simulink model "Prediction_and_cost_function_FCS_MPC_6Phase_PMSM"  (R2022a)
settings: Solver=FixedStepDiscrete  StartTime=0.0  StopTime=10.0  RelTol=1e-3
values from neighbouring files (symbols this model uses):
  f_c = 100000    [MPC_params.m]
  L_d = 2e-3    (= 0.002)    [MPC_params.m]
  L_q = 6.4e-3    (= 0.0064)    [MPC_params.m]
  L_x = 3e-3    (= 0.003)    [MPC_params.m]
  L_y = L_x    (= 0.003)    [MPC_params.m]
  p = 5    [MPC_params.m]
  psi_pm = 0.19    [MPC_params.m]
  R_ph = 0.19    [MPC_params.m]
libraries: hdlsllib x5
settings Model: DataTypeOverride=Off  Creator=Andre Merx  LastModifiedBy=Andre Merx
settings SolverCC: AlgebraicLoopSolver=TrustRegion
settings DataIOCC: LimitDataPoints=on  SaveOutput=off  SaveTime=off
settings OptimizationCC: BlockReduction=off  ConditionallyExecuteInputs=off  DefaultParameterBehavior=Inlined  LifeSpan=inf
settings DebuggingCC: AlgebraicLoopMsg=error  SingleTaskRateTransMsg=error  UnconnectedInputMsg=warning  UnconnectedOutputMsg=warning  UnconnectedLineMsg=warning  AllowSymbolicDim=off  StrictBusMsg=ErrorOnBusTreatedAsVector  SFUnexpectedBacktrackingDiag=warning  SFNoUnconditionalDefaultTransitionDiag=warning  SFExecutionAtInitializationDiag=none  SFMachineParentedDataDiag=warning  ArithmeticOperatorsInVariantConditions=warning
settings HardwareCC: ProdBitPerPointer=32  ProdBitPerSizeT=32  ProdBitPerPtrDiffT=32  ProdLargestAtomicFloat=None  ProdIntDivRoundTo=Undefined  ProdEndianess=Unspecified  ProdWordSize=32  ProdHWDeviceType=ASIC/FPGA->ASIC/FPGA  ProdEqTarget=off
settings SFSimCC: SimUseLocalCustomCode=off  CustomCodeUndefinedFunction=UseInterfaceOnly
settings RTWCC: RTWUseLocalCustomCode=off
settings CodeAppCC: StateflowObjectComments=on
settings GRTTargetCC: TargetLangStandard=C89/C90 (ANSI)
settings ConfigComp: CovScope=ReferencedModels  CovMetricSettings=dw  CovSaveCumulativeToWorkspaceVar=on  CovSaveSingleToWorkspaceVar=on  CovExternalEMLEnable=off  CovSFcnEnable=off

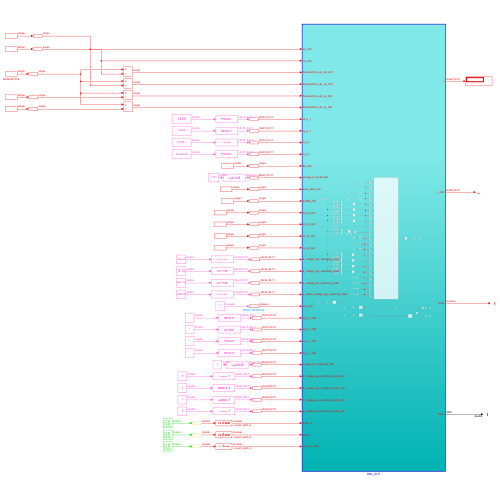
[thumbnail: Simulink's stored preview of the top-level diagram]
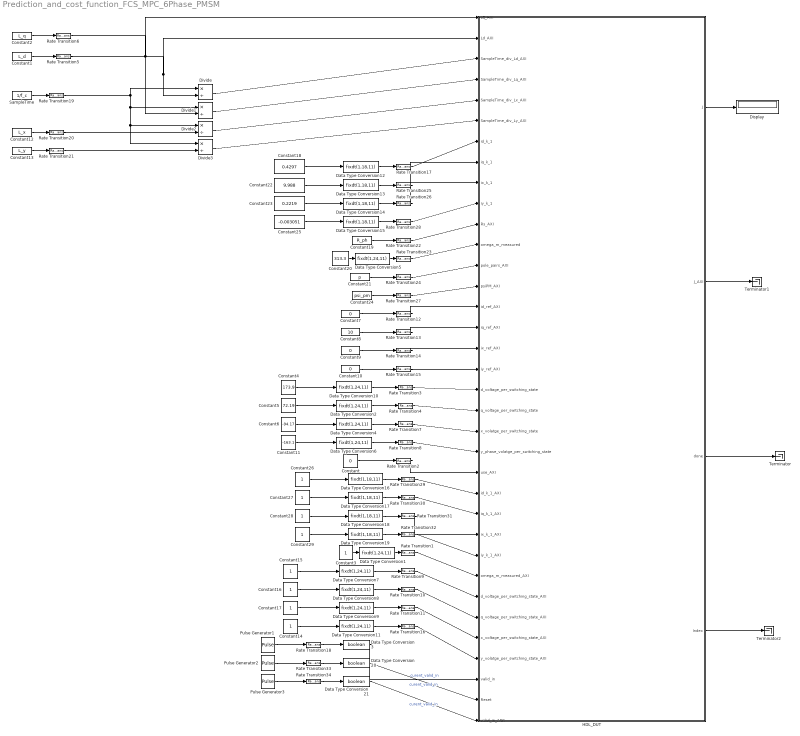
== system Prediction_and_cost_function_FCS_MPC_6Phase_PMSM ==
  Constant : Constant  Value=0  OutDataTypeStr=boolean
  Constant1 : Constant  Value=L_d  OutDataTypeStr=single  SampleTime=-1
  Constant10 : Constant  Value=0  OutDataTypeStr=single  SampleTime=-1
  Constant11 : Constant  Value=-163.1
  Constant12 : Constant  Value=L_x  OutDataTypeStr=single  SampleTime=-1
  Constant13 : Constant  Value=L_y  OutDataTypeStr=single  SampleTime=-1
  Constant{3,14..17,26..29} (9 alike) : Constant
  Constant18 : Constant  Value=0.4297
  Constant19 : Constant  Value=R_ph  OutDataTypeStr=single  SampleTime=-1
  Constant2 : Constant  Value=L_q  OutDataTypeStr=single  SampleTime=-1
  Constant20 : Constant  Value=313.3
  Constant21 : Constant  Value=p  OutDataTypeStr=single  SampleTime=-1
  Constant22 : Constant  Value=9.988
  Constant23 : Constant  Value=0.2219
  Constant24 : Constant  Value=psi_pm  OutDataTypeStr=single  SampleTime=-1
  Constant25 : Constant  Value=-0.003051
  Constant4 : Constant  Value=173.9
  Constant5 : Constant  Value=72.19
  Constant6 : Constant  Value=-94.17
  Constant7 : Constant  Value=0  OutDataTypeStr=single  SampleTime=-1
  Constant8 : Constant  Value=10  OutDataTypeStr=single  SampleTime=-1
  Constant9 : Constant  Value=0  OutDataTypeStr=single  SampleTime=-1
  Data Type Conversion{1..2,4..11} (10 alike) : DataTypeConversion  OutDataTypeStr=fixdt(1,24,11)  SaturateOnIntegerOverflow=off  RndMeth=Floor
  Data Type Conversion{12..19} (8 alike) : DataTypeConversion  OutDataTypeStr=fixdt(1,18,11)  SaturateOnIntegerOverflow=off  RndMeth=Floor
  Data Type Conversion20 : DataTypeConversion  OutDataTypeStr=boolean  SaturateOnIntegerOverflow=off  RndMeth=Floor
  Data Type Conversion21 : DataTypeConversion  OutDataTypeStr=boolean  SaturateOnIntegerOverflow=off  RndMeth=Floor
  Data Type Conversion3 : DataTypeConversion  OutDataTypeStr=boolean  SaturateOnIntegerOverflow=off  RndMeth=Floor
  Display : Display
  Divide{,1..3} (4 alike) : Product  Inputs=*/  RndMeth=Zero  SaturateOnIntegerOverflow=on
  HDL_DUT : Subsystem  TreatAsAtomicUnit=on
  Pulse Generator1 : DiscretePulseGenerator  PulseType=Time based  Period=1/f_c
  Pulse Generator2 : DiscretePulseGenerator  PulseType=Time based  Period=1/f_c
  Pulse Generator3 : DiscretePulseGenerator  PulseType=Time based  Period=1/f_c
  Rate Transition{1..34} (34 alike) : RateTransition  OutPortSampleTime=Rt
  SampleTime : Constant  Value=1/f_c  OutDataTypeStr=single  SampleTime=-1
  Terminator : Terminator
  Terminator1 : Terminator
  Terminator2 : Terminator
  wires:
  Constant7/1 -> Rate Transition12/1
  Constant9/1 -> Rate Transition14/1
  Constant8/1 -> Rate Transition13/1
  Constant10/1 -> Rate Transition15/1
  Rate Transition24/1 -> HDL_DUT/13(pole_pairs_AXI)
  Rate Transition27/1 -> HDL_DUT/14(psiPM_AXI)
  Data Type Conversion5/1 -> Rate Transition23/1
  Constant21/1 -> Rate Transition24/1
  Constant24/1 -> Rate Transition27/1
  Rate Transition23/1 -> HDL_DUT/12(omega_m_measured)
  Rate Transition22/1 -> HDL_DUT/11(Rs_AXI)
  Constant20/1 -> Data Type Conversion5/1
  Constant19/1 -> Rate Transition22/1
  Rate Transition6/1 -> HDL_DUT/1(Lq_AXI), Divide1/2
  Rate Transition5/1 -> HDL_DUT/2(Ld_AXI), Divide/2
  Constant1/1 -> Rate Transition5/1
  Constant13/1 -> Rate Transition21/1
  Rate Transition21/1 -> Divide3/2
  Constant2/1 -> Rate Transition6/1
  Constant12/1 -> Rate Transition20/1
  Rate Transition19/1 -> Divide1/1, Divide3/1, Divide2/1, Divide/1
  Rate Transition20/1 -> Divide2/2
  SampleTime/1 -> Rate Transition19/1
  Divide/1 -> HDL_DUT/3(SampleTime_div_Ld_AXI)
  Divide1/1 -> HDL_DUT/4(SampleTime_div_Lq_AXI)
  Divide2/1 -> HDL_DUT/5(SampleTime_div_Lx_AXI)
  Divide3/1 -> HDL_DUT/6(SampleTime_div_Ly_AXI)
  Rate Transition12/1 -> HDL_DUT/15(id_ref_AXI)
  Rate Transition13/1 -> HDL_DUT/16(iq_ref_AXI)
  Rate Transition14/1 -> HDL_DUT/17(ix_ref_AXI)
  Rate Transition15/1 -> HDL_DUT/18(iy_ref_AXI)
  HDL_DUT/3(done) -> Terminator/1
  HDL_DUT/2(J_AXI) -> Terminator1/1
  HDL_DUT/1(J) -> Display/1
  Data Type Conversion3/1 -> HDL_DUT/33(valid_in)  "curent_valid_in"
  Rate Transition18/1 -> Data Type Conversion3/1
  Pulse Generator1/1 -> Rate Transition18/1
  Constant3/1 -> Data Type Conversion1/1
  Data Type Conversion1/1 -> Rate Transition1/1
  Rate Transition1/1 -> HDL_DUT/28(omega_m_measured_AXI)
  Constant/1 -> Rate Transition2/1
  Rate Transition2/1 -> HDL_DUT/23(use_AXI)
  Data Type Conversion10/1 -> Rate Transition3/1
  Rate Transition3/1 -> HDL_DUT/19(d_voltage_per_switching_state)
  Data Type Conversion2/1 -> Rate Transition4/1
  Rate Transition4/1 -> HDL_DUT/20(q_voltage_per_switching_state)
  Data Type Conversion4/1 -> Rate Transition7/1
  Rate Transition7/1 -> HDL_DUT/21(x_volatge_per_switching_state)
  Data Type Conversion6/1 -> Rate Transition8/1
  Rate Transition8/1 -> HDL_DUT/22(y_phase_volatge_per_switching_state)
  Constant4/1 -> Data Type Conversion10/1
  Constant5/1 -> Data Type Conversion2/1
  Constant6/1 -> Data Type Conversion4/1
  Constant11/1 -> Data Type Conversion6/1
  Constant17/1 -> Data Type Conversion9/1
  Constant15/1 -> Data Type Conversion7/1
  Constant14/1 -> Data Type Conversion11/1
  Rate Transition16/1 -> HDL_DUT/32(y_volatge_per_switching_state_AXI)
  Constant16/1 -> Data Type Conversion8/1
  Rate Transition10/1 -> HDL_DUT/30(q_voltage_per_switching_state_AXI)
  Rate Transition11/1 -> HDL_DUT/31(x_voltage_per_switching_state_AXI)
  Data Type Conversion8/1 -> Rate Transition10/1
  Data Type Conversion9/1 -> Rate Transition11/1
  Data Type Conversion11/1 -> Rate Transition16/1
  Data Type Conversion7/1 -> Rate Transition9/1
  Rate Transition9/1 -> HDL_DUT/29(d_voltage_per_switching_state_AXI)
  Data Type Conversion12/1 -> Rate Transition17/1
  Rate Transition17/1 -> HDL_DUT/7(id_k_1)
  Data Type Conversion13/1 -> Rate Transition25/1
  Rate Transition25/1 -> HDL_DUT/8(iq_k_1)
  Data Type Conversion14/1 -> Rate Transition26/1
  Rate Transition26/1 -> HDL_DUT/9(ix_k_1)
  Data Type Conversion15/1 -> Rate Transition28/1
  Rate Transition28/1 -> HDL_DUT/10(iy_k_1)
  Constant18/1 -> Data Type Conversion12/1
  Constant22/1 -> Data Type Conversion13/1
  Constant23/1 -> Data Type Conversion14/1
  Constant25/1 -> Data Type Conversion15/1
  Rate Transition32/1 -> HDL_DUT/27(iy_k_1_AXI)
  Data Type Conversion17/1 -> Rate Transition30/1
  Constant29/1 -> Data Type Conversion19/1
  Constant26/1 -> Data Type Conversion16/1
  Data Type Conversion16/1 -> Rate Transition29/1
  Data Type Conversion18/1 -> Rate Transition31/1
  Constant28/1 -> Data Type Conversion18/1
  Data Type Conversion19/1 -> Rate Transition32/1
  Rate Transition30/1 -> HDL_DUT/25(iq_k_1_AXI)
  Constant27/1 -> Data Type Conversion17/1
  Rate Transition29/1 -> HDL_DUT/24(id_k_1_AXI)
  Rate Transition31/1 -> HDL_DUT/26(ix_k_1_AXI)
  Pulse Generator2/1 -> Rate Transition33/1
  Data Type Conversion20/1 -> HDL_DUT/34(Reset)  "curent_valid_in"
  Rate Transition33/1 -> Data Type Conversion20/1
  Pulse Generator3/1 -> Rate Transition34/1
  Data Type Conversion21/1 -> HDL_DUT/35(valid_in_ADC)  "curent_valid_in"
  Rate Transition34/1 -> Data Type Conversion21/1
  HDL_DUT/4(Index) -> Terminator2/1

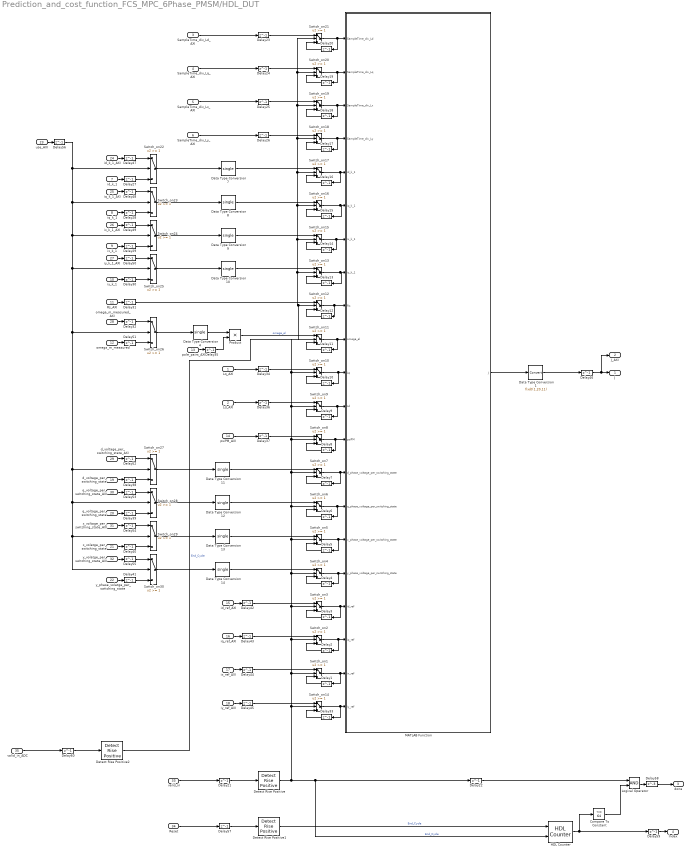
== system Prediction_and_cost_function_FCS_MPC_6Phase_PMSM/HDL_DUT ==
  Lq_AXI : Inport
  Ld_AXI : Inport  Port=2
  SampleTime_div_Ld_AXI : Inport  Port=3
  SampleTime_div_Lq_AXI : Inport  Port=4
  SampleTime_div_Lx_AXI : Inport  Port=5
  SampleTime_div_Ly_AXI : Inport  Port=6
  id_k_1 : Inport  Port=7
  iq_k_1 : Inport  Port=8
  ix_k_1 : Inport  Port=9
  iy_k_1 : Inport  Port=10
  Rs_AXI : Inport  Port=11
  omega_m_measured : Inport  Port=12
  pole_pairs_AXI : Inport  Port=13
  psiPM_AXI : Inport  Port=14
  id_ref_AXI : Inport  Port=15
  iq_ref_AXI : Inport  Port=16
  ix_ref_AXI : Inport  Port=17
  iy_ref_AXI : Inport  Port=18
  d_voltage_per_switching_state : Inport  Port=19
  q_voltage_per_switching_state : Inport  Port=20
  x_volatge_per_switching_state : Inport  Port=21
  y_phase_volatge_per_switching_state : Inport  Port=22
  use_AXI : Inport  Port=23
  id_k_1_AXI : Inport  Port=24
  iq_k_1_AXI : Inport  Port=25
  ix_k_1_AXI : Inport  Port=26
  iy_k_1_AXI : Inport  Port=27
  omega_m_measured_AXI : Inport  Port=28
  d_voltage_per_switching_state_AXI : Inport  Port=29
  q_voltage_per_switching_state_AXI : Inport  Port=30
  x_voltage_per_switching_state_AXI : Inport  Port=31
  y_volatge_per_switching_state_AXI : Inport  Port=32
  valid_in : Inport  Port=33
  Reset : Inport  Port=34
  valid_in_ADC : Inport  Port=35
  Compare To Constant : hdlsllib/Logic and Bit Operations/Compare To Constant  relop=<=  const=64  OutDataTypeStr=boolean
      settings: SourceProductBaseCode=SL
  Data Type Conversion1 : DataTypeConversion  OutDataTypeStr=fixdt(1,20,11)  RndMeth=Nearest  SaturateOnIntegerOverflow=off
  Data Type Conversion{4,7..14} (9 alike) : DataTypeConversion  OutDataTypeStr=single  RndMeth=Nearest  SaturateOnIntegerOverflow=off
  Delay{1..57,59..60} (59 alike) : Delay  DelayLength=1
  Delay58 : Delay  DelayLength=3
  Detect Rise Positive : hdlsllib/Logic and Bit Operations/Detect Rise Positive  vinit=0  OutDataTypeStr=boolean
      settings: SourceProductBaseCode=SL
  Detect Rise Positive1 : hdlsllib/Logic and Bit Operations/Detect Rise Positive  vinit=0  OutDataTypeStr=boolean
      settings: SourceProductBaseCode=SL
  Detect Rise Positive2 : hdlsllib/Logic and Bit Operations/Detect Rise Positive  vinit=0  OutDataTypeStr=boolean
      settings: SourceProductBaseCode=SL
  HDL Counter : hdlsllib/Sources/HDL Counter  CountType=Free running  CountInit=0  CountStep=1  CountMax=25  CountFromType=Initial value  CountFrom=0  CountResetPort=on  CountLoadPort=off  CountEnbPort=on  CountDirPort=off  CountHitOutputPort=off  CountDataType=Signed  CountWordLen=32  CountFracLen=0  CountSampTime=1
  Logical Operator : Logic  AllPortsSameDT=off  OutDataTypeStr=boolean
  MATLAB Function : MATLAB Function  TreatAsAtomicUnit=on
  Product : Product  Inputs=**
  Switch_on{1..21} (21 alike) : Switch  Threshold=1  OutDataTypeStr=single  RndMeth=Simplest  SaturateOnIntegerOverflow=off  InputSameDT=off
  Switch_on{22..30} (9 alike) : Switch  Threshold=1  OutDataTypeStr=Inherit: Inherit via back propagation  RndMeth=Simplest  SaturateOnIntegerOverflow=off  InputSameDT=off
  J : Outport
  J_AXI : Outport  Port=2
  done : Outport  Port=3
  Index : Outport  Port=4
  wires:
  Switch_on12/1 -> Delay12/1, MATLAB Function/9(Rs)
  Rs_AXI/1 -> Delay31/1
  Delay31/1 -> Switch_on12/1
  Delay23/1 -> Switch_on21/1
  Delay46/1 -> J_AXI/1, J/1
  Delay28/1 -> Switch_on23/3
  Delay3/1 -> Switch_on3/3
  Delay10/1 -> Switch_on10/3
  Delay43/1 -> Switch_on2/1
  Switch_on5/1 -> MATLAB Function/16(x_phase_voltage_per_switching_state), Delay5/1
  Delay40/1 -> Switch_on29/3
  Delay17/1 -> Switch_on18/3
  Switch_on10/1 -> MATLAB Function/11(Lq), Delay10/1
  Delay11/1 -> Switch_on11/3
  Delay29/1 -> Switch_on24/3
  Delay38/1 -> Switch_on27/3
  Switch_on6/1 -> Delay6/1, MATLAB Function/15(q_phase_voltage_per_switching_state)
  Delay24/1 -> Switch_on20/1
  Delay36/1 -> Switch_on9/1
  Delay37/1 -> Switch_on8/1
  Delay1/1 -> Switch_on1/3
  Delay42/1 -> Switch_on3/1
  Product/1 -> Switch_on11/1  "omega_el"
  valid_in/1 -> Delay21/1
  y_phase_volatge_per_switching_state/1 -> Delay41/1
  Delay27/1 -> Switch_on22/3
  Delay30/1 -> Switch_on25/3
  Delay9/1 -> Switch_on9/3
  Data Type Conversion4/1 -> Product/1
  iy_k_1/1 -> Delay30/1
  Delay20/1 -> Switch_on21/3
  Delay35/1 -> Product/2
  pole_pairs_AXI/1 -> Delay35/1
  omega_m_measured/1 -> Delay51/1
  Switch_on18/1 -> Delay17/1, MATLAB Function/4(SampleTime_div_Ly)
  Delay19/1 -> Switch_on20/3
  Delay13/1 -> Switch_on13/3
  Delay22/1 -> Logical Operator/1
  Delay7/1 -> Switch_on7/3
  Delay4/1 -> Switch_on4/3
  Switch_on15/1 -> Delay14/1, MATLAB Function/7(ix_k_1)
  Delay18/1 -> Switch_on19/3
  Lq_AXI/1 -> Delay34/1
  Switch_on19/1 -> Delay18/1, MATLAB Function/3(SampleTime_div_Lx)
  Switch_on20/1 -> Delay19/1, MATLAB Function/2(SampleTime_div_Lq)
  Switch_on13/1 -> Delay13/1, MATLAB Function/8(iy_k_1)
  ix_k_1/1 -> Delay29/1
  Delay45/1 -> Switch_on14/1
  Delay2/1 -> Switch_on2/3
  Delay16/1 -> Switch_on17/3
  Switch_on17/1 -> Delay16/1, MATLAB Function/5(id_k_1)
  iq_k_1/1 -> Delay28/1
  Delay15/1 -> Switch_on16/3
  Switch_on16/1 -> Delay15/1, MATLAB Function/6(iq_k_1)
  d_voltage_per_switching_state/1 -> Delay38/1
  iq_ref_AXI/1 -> Delay43/1
  Switch_on7/1 -> Delay7/1, MATLAB Function/14(d_phase_voltage_per_switching_state)
  Switch_on11/1 -> Delay11/1, MATLAB Function/10(omega_el)
  Delay33/1 -> Switch_on14/3
  Ld_AXI/1 -> Delay36/1
  Delay25/1 -> Switch_on19/1
  psiPM_AXI/1 -> Delay37/1
  Switch_on14/1 -> Delay33/1, MATLAB Function/21(iy_ref)
  Delay12/1 -> Switch_on12/3
  Delay6/1 -> Switch_on6/3
  Delay21/1 -> Detect Rise Positive/1
  Switch_on3/1 -> Delay3/1, MATLAB Function/18(id_ref)
  Switch_on21/1 -> Delay20/1, MATLAB Function/1(SampleTime_div_Ld)
  Switch_on2/1 -> MATLAB Function/19(iq_ref), Delay2/1
  MATLAB Function/1(J) -> Data Type Conversion1/1
  Delay34/1 -> Switch_on10/1
  Detect Rise Positive/1 -> HDL Counter/2, Delay22/1, Switch_on14/2, Switch_on1/2, Switch_on5/2, Switch_on8/2, Switch_on9/2, Switch_on12/2, Switch_on13/2, Switch_on21/2, Switch_on20/2, Switch_on19/2, Switch_on18/2, Switch_on17/2, Switch_on16/2, Switch_on15/2, Switch_on10/2, Switch_on7/2, Switch_on6/2, Switch_on4/2, Switch_on3/2, Switch_on2/2  "End_Cycle"
  q_voltage_per_switching_state/1 -> Delay39/1
  iy_ref_AXI/1 -> Delay45/1
  Switch_on1/1 -> Delay1/1, MATLAB Function/20(ix_ref)
  id_k_1/1 -> Delay27/1
  ix_ref_AXI/1 -> Delay44/1
  Switch_on9/1 -> MATLAB Function/12(Ld), Delay9/1
  Delay39/1 -> Switch_on28/3
  Delay26/1 -> Switch_on18/1
  x_volatge_per_switching_state/1 -> Delay40/1
  Delay14/1 -> Switch_on15/3
  Delay41/1 -> Switch_on30/3
  Switch_on4/1 -> MATLAB Function/17(y_phase_voltage_per_switching_state), Delay4/1
  id_ref_AXI/1 -> Delay42/1
  Delay44/1 -> Switch_on1/1
  Switch_on8/1 -> Delay8/1, MATLAB Function/13(psiPM)
  Delay5/1 -> Switch_on5/3
  Delay8/1 -> Switch_on8/3
  Switch_on22/1 -> Data Type Conversion7/1
  Delay47/1 -> Switch_on22/1
  id_k_1_AXI/1 -> Delay47/1
  Switch_on23/1 -> Data Type Conversion8/1
  Delay48/1 -> Switch_on23/1
  iq_k_1_AXI/1 -> Delay48/1
  Switch_on24/1 -> Data Type Conversion9/1
  ix_k_1_AXI/1 -> Delay49/1
  Delay49/1 -> Switch_on24/1
  Switch_on25/1 -> Data Type Conversion10/1
  iy_k_1_AXI/1 -> Delay50/1
  Delay50/1 -> Switch_on25/1
  Delay51/1 -> Switch_on26/3
  Switch_on26/1 -> Data Type Conversion4/1
  omega_m_measured_AXI/1 -> Delay32/1
  Delay32/1 -> Switch_on26/1
  Switch_on27/1 -> Data Type Conversion11/1
  Delay52/1 -> Switch_on27/1
  d_voltage_per_switching_state_AXI/1 -> Delay52/1
  Switch_on28/1 -> Data Type Conversion12/1
  q_voltage_per_switching_state_AXI/1 -> Delay53/1
  Delay53/1 -> Switch_on28/1
  Switch_on29/1 -> Data Type Conversion13/1
  x_voltage_per_switching_state_AXI/1 -> Delay54/1
  Delay54/1 -> Switch_on29/1
  Switch_on30/1 -> Data Type Conversion14/1
  Delay55/1 -> Switch_on30/1
  y_volatge_per_switching_state_AXI/1 -> Delay55/1
  use_AXI/1 -> Delay56/1
  Delay56/1 -> Switch_on22/2, Switch_on29/2, Switch_on30/2, Switch_on28/2, Switch_on27/2, Switch_on26/2, Switch_on25/2, Switch_on24/2, Switch_on23/2
  Data Type Conversion1/1 -> Delay46/1
  SampleTime_div_Ld_AXI/1 -> Delay23/1
  SampleTime_div_Lq_AXI/1 -> Delay24/1
  SampleTime_div_Lx_AXI/1 -> Delay25/1
  SampleTime_div_Ly_AXI/1 -> Delay26/1
  Data Type Conversion7/1 -> Switch_on17/1
  Data Type Conversion8/1 -> Switch_on16/1
  Data Type Conversion9/1 -> Switch_on15/1
  Data Type Conversion10/1 -> Switch_on13/1
  Data Type Conversion11/1 -> Switch_on7/1
  Data Type Conversion12/1 -> Switch_on6/1
  Data Type Conversion13/1 -> Switch_on5/1
  Data Type Conversion14/1 -> Switch_on4/1
  HDL Counter/1 -> Compare To Constant/1, Delay59/1
  Reset/1 -> Delay57/1
  Detect Rise Positive1/1 -> HDL Counter/1  "End_Cycle"
  Delay57/1 -> Detect Rise Positive1/1
  Delay59/1 -> Index/1
  Logical Operator/1 -> Delay58/1
  Delay58/1 -> done/1
  Compare To Constant/1 -> Logical Operator/2
  valid_in_ADC/1 -> Delay60/1
  Delay60/1 -> Detect Rise Positive2/1
  Detect Rise Positive2/1 -> Switch_on11/2  "End_Cycle"

== matlab function Prediction_and_cost_function_FCS_MPC_6Phase_PMSM/HDL_DUT/MATLAB Function ==
  data: SampleTime_div_Ld input; J output; SampleTime_div_Lq input; SampleTime_div_Lx input; SampleTime_div_Ly input; id_k_1 input; iq_k_1 input; ix_k_1 input; iy_k_1 input; Rs input; omega_el input; Lq input; Ld input; psiPM input; d_phase_voltage_per_switching_state input; q_phase_voltage_per_switching_state input; x_phase_voltage_per_switching_state input; y_phase_voltage_per_switching_state input; id_ref input; iq_ref input; ix_ref input; iy_ref input
function J = fcn(SampleTime_div_Ld, SampleTime_div_Lq, SampleTime_div_Lx, SampleTime_div_Ly, id_k_1, iq_k_1, ix_k_1, iy_k_1, Rs, omega_el, Lq, Ld, psiPM, d_phase_voltage_per_switching_state, q_phase_voltage_per_switching_state, x_phase_voltage_per_switching_state, y_phase_voltage_per_switching_state, id_ref, iq_ref, ix_ref, iy_ref)
     
        % Prediction of the d-, q-, x-, y-currents of the 6-Phase-PMSM with the finite control set 
        id_k_2 = single(SampleTime_div_Ld*(d_phase_voltage_per_switching_state-id_k_1*Rs+omega_el*Lq*iq_k_1)+id_k_1);
        iq_k_2 = single(SampleTime_div_Lq*(q_phase_voltage_per_switching_state-iq_k_1*Rs-omega_el*(psiPM+id_k_1*Ld))+iq_k_1);
        ix_k_2 = single(SampleTime_div_Lx*(x_phase_voltage_per_switching_state-ix_k_1*Rs)+ix_k_1);
        iy_k_2 = single(SampleTime_div_Ly*(y_phase_voltage_per_switching_state-iy_k_1*Rs)+iy_k_1);
        
        % Calculation of the cost function
        J = single((id_ref-id_k_2)^2+(iq_ref-iq_k_2)^2+(ix_ref-ix_k_2)^2+(iy_ref-iy_k_2)^2);

end
